simulink model "simscape_robot_delta_v9"  (R2024b)
settings: Solver=FixedStepAuto  StartTime=0.0  StopTime=20.0  FixedStep=1e-6  RelTol=1e-3
model workspace (MAT data in the model file):
  Ts = 1e-06
  kd1 = 14
  kd2 = 13.6
  kd3 = 37.9
  ki1 = 39
  ki2 = 36
  ki3 = 11.6
  kp1 = 12.6
  kp2 = 12.2
  kp3 = 14.4
values from neighbouring files (symbols this model uses):
  N = floor(size(err,1)/window)    [grafica_error.m]
undefined symbols (not defined in the file or in its folder): DiscIntNeverNeededParam, X, Y, Z
libraries: sm_lib x81, nesl_utility x7, spsUniversalBridgeLib x6, spsCurrentMeasurementLib x6, spsDCVoltageSourceLib x3, spsStepperMotorLib x3, spspowerguiLib x1
(part 1 of 3)
settings Model: Creator=rodri  LastModifiedBy=rodri

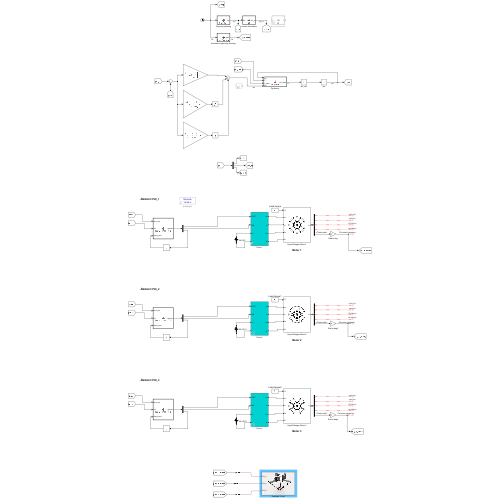
[thumbnail: Simulink's stored preview of the top-level diagram]
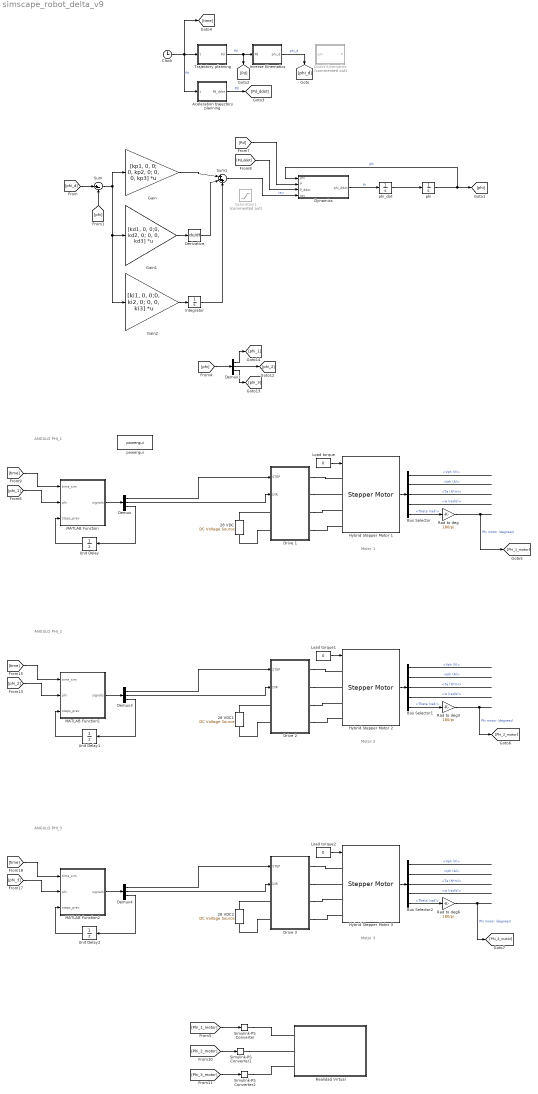
== system simscape_robot_delta_v9 ==
  note: Motor 3
  note: ÁNGULO PHI_1
  note: Motor 1
  note: ÁNGULO PHI_2
  note: ÁNGULO PHI_3
  note: Motor 2
  28 VDC : spsDCVoltageSourceLib/DC Voltage Source  Amplitude=28  Measurements=None
  28 VDC1 : spsDCVoltageSourceLib/DC Voltage Source  Amplitude=28  Measurements=None
  28 VDC2 : spsDCVoltageSourceLib/DC Voltage Source  Amplitude=28  Measurements=None
  Aceleration trajectory planning : MATLAB Function  TreatAsAtomicUnit=on
  Bus Selector : BusSelector  OutputSignals=Vph (V),Iph (A),Te (N*m),w (rad/s),Theta (rad)
  Bus Selector1 : BusSelector  OutputSignals=Vph (V),Iph (A),Te (N*m),w (rad/s),Theta (rad)
  Bus Selector2 : BusSelector  OutputSignals=Vph (V),Iph (A),Te (N*m),w (rad/s),Theta (rad)
  Clock : Clock
  Demux{,1,3..4} (4 alike) : Demux  Outputs=3
  Derivative : Derivative
  Direct Kinematics : MATLAB Function  Commented=on  TreatAsAtomicUnit=on
  Drive 1 : Subsystem  mask{Iref=2, step=500, Ts=Ts}
      mask prompts: Iref "Phase current (A)"; step "Stepping rate (step/s)"; Ts "Sampling time (s)"
      mask init:
      | Nstep=round(1/step/Ts);
  Drive 2 : Subsystem  mask{Iref=2, step=500, Ts=Ts}
      mask prompts: Iref "Phase current (A)"; step "Stepping rate (step/s)"; Ts "Sampling time (s)"
      mask init:
      | Nstep=round(1/step/Ts);
  Drive 3 : Subsystem  mask{Iref=2, step=500, Ts=Ts}
      mask prompts: Iref "Phase current (A)"; step "Stepping rate (step/s)"; Ts "Sampling time (s)"
      mask init:
      | Nstep=round(1/step/Ts);
  Dynamics : MATLAB Function  TreatAsAtomicUnit=on
  Gain : Gain  Gain=[kp1, 0, 0; 0, kp2, 0; 0, 0, kp3]  Multiplication=Matrix(K*u)
  Gain1 : Gain  Gain=[kd1, 0, 0;0, kd2, 0; 0, 0, kd3]  Multiplication=Matrix(K*u)
  Gain2 : Gain  Gain=[ki1, 0, 0;0, ki2, 0; 0, 0, ki3]  Multiplication=Matrix(K*u)
  Hybrid Stepper Motor 1 : spsStepperMotorLib/Stepper Motor  MotorType=Permanent-magnet / Hybrid  NumberOfPhases_1=2  NumberOfPhases_2=3  PresetModel_1=<empty>  PresetModel_2=<empty>  L=1.4e-3  Lmax=10e-3  Lmin=2e-3  R=0.7  Step_angle=1.8  Psim=0.005  Tdm=0.002  J=1.2e-7  B=1e-7*1000  w0=0  pos0=0  TsPowergui=0  TsBlock=-1
  Hybrid Stepper Motor 2 : spsStepperMotorLib/Stepper Motor  MotorType=Permanent-magnet / Hybrid  NumberOfPhases_1=2  NumberOfPhases_2=3  PresetModel_1=<empty>  PresetModel_2=<empty>  L=1.4e-3  Lmax=10e-3  Lmin=2e-3  R=0.7  Step_angle=1.8  Psim=0.005  Tdm=0.002  J=1.2e-7  B=1e-7*1000  w0=0  pos0=0  TsPowergui=0  TsBlock=-1
  Hybrid Stepper Motor 3 : spsStepperMotorLib/Stepper Motor  MotorType=Permanent-magnet / Hybrid  NumberOfPhases_1=2  NumberOfPhases_2=3  PresetModel_1=<empty>  PresetModel_2=<empty>  L=1.4e-3  Lmax=10e-3  Lmin=2e-3  R=0.7  Step_angle=1.8  Psim=0.005  Tdm=0.002  J=1.2e-7  B=1e-7*1000  w0=0  pos0=0  TsPowergui=0  TsBlock=-1
  Integrator : Integrator  InitialCondition=[0;0;0]
  Inverse Kinematics : MATLAB Function  TreatAsAtomicUnit=on
  Load torque : Constant  Value=0
  Load torque1 : Constant  Value=0
  Load torque2 : Constant  Value=0
  MATLAB Function : MATLAB Function  TreatAsAtomicUnit=on
  MATLAB Function1 : MATLAB Function  TreatAsAtomicUnit=on
  MATLAB Function2 : MATLAB Function  TreatAsAtomicUnit=on
  Rad to deg : Gain  Gain=180/pi
  Rad to deg3 : Gain  Gain=180/pi
  Rad to deg6 : Gain  Gain=180/pi
  Realidad Virtual : Subsystem
      mask Display: image('robot_delta_azucena.png');
  Saturation1 : Saturate  Commented=on  UpperLimit=19.8  LowerLimit=-19.8
  Simulink-PS Converter : nesl_utility/Simulink-PS Converter  PhysicalDomain=network_engine_domain  SubClassName=ps_input  LeftPortType=input  RightPortType=output  PseudoPeriodic=off  Frequencies=[]  NoiseDistribution=none  NoiseParameters=[]  Unit=deg  AffineConversion=off  FilteringAndDerivatives=filter  SimscapeFilterOrder=2  InputFilterTimeConstant=0.001  UdotUserProvided=0
  Simulink-PS Converter1 : nesl_utility/Simulink-PS Converter  PhysicalDomain=network_engine_domain  SubClassName=ps_input  LeftPortType=input  RightPortType=output  PseudoPeriodic=off  Frequencies=[]  NoiseDistribution=none  NoiseParameters=[]  Unit=deg  AffineConversion=off  FilteringAndDerivatives=filter  SimscapeFilterOrder=2  InputFilterTimeConstant=0.001  UdotUserProvided=0
  Simulink-PS Converter2 : nesl_utility/Simulink-PS Converter  PhysicalDomain=network_engine_domain  SubClassName=ps_input  LeftPortType=input  RightPortType=output  PseudoPeriodic=off  Frequencies=[]  NoiseDistribution=none  NoiseParameters=[]  Unit=deg  AffineConversion=off  FilteringAndDerivatives=filter  SimscapeFilterOrder=2  InputFilterTimeConstant=0.001  UdotUserProvided=0
  Sum : Sum  Inputs=|+-
  Sum1 : Sum  Inputs=|+++
  Trajectory planning : MATLAB Function  TreatAsAtomicUnit=on
  Unit Delay : UnitDelay  SampleTime=-1  HasFrameUpgradeWarning=on
  Unit Delay1 : UnitDelay  SampleTime=-1  HasFrameUpgradeWarning=on
  Unit Delay2 : UnitDelay  SampleTime=-1  HasFrameUpgradeWarning=on
  phi : Integrator  InitialCondition=[0;0;0]
  phi_dot : Integrator  InitialCondition=[0;0;0]
  powergui : spspowerguiLib/powergui  SimulationMode=Discrete  SampleTime=Ts  frequency=60  Iterations=50  frequencyindice=0  Pbase=100e6  ErrMax=1e-4  UnitsV=kV  UnitsW=MW  buscounter=0  FunctionMessages=off  echomessages=off  EnableUseOfTLC=off  CurrentSourceSwitches=off  DisableSnubberDevices=off  DisableRonSwitches=off  DisableVfSwitches=off  DisplayEquations=off  AutomaticDiscreteSolvers=off  SolverType=Tustin/Backward Euler (TBE)  Interpol=off  ExternalGateDelay=off  methode=off  Ts=0  x0status=blocks  SPID=off  SwTol=0  HookPort=off  NonlinearTolerance=1e-4  nMaxIteration=100  ContinueOnMaxIteration=off  RestoreLinks=warning  ResistiveCurrentMeasurement=off  Frange=[0:2:500]  Ylog=off  Xlog=on  ShowGrid=off  save=off  variable=ZData  structure=0  ZoomFFT=on  StartTime=0.0  cycles=1  DisplayStyle=1  fundamental=60  FreqAxis=off  MaxFrequency=1000  frequencyindicesteady=1  RmsSteady=1  display=off
  wires:
  Sum/1 -> Gain2/1, Gain1/1, Gain/1
  Gain/1 -> Sum1/1
  Derivative/1 -> Sum1/2
  [Pd] -> Dynamics/2(P)
  Clock/1 -> [time], Aceleration trajectory planning/1(t), Trajectory planning/1(t)  "Pd"
  phi/1 -> Dynamics/1(phi), [phi]  "phi"
  Integrator/1 -> Sum1/3
  [Pd_ddot] -> Dynamics/3(P_ddot)
  Sum1/1 -> Dynamics/4(tau)  "tau"
  Gain1/1 -> Derivative/1
  [phi_d] -> Sum/1
  Trajectory planning/1(Pd) -> Inverse Kinematics/1(Pd), [Pd]  "Pd"
  Dynamics/1(phi_ddot) -> phi_dot/1  "Pr"
  Gain2/1 -> Integrator/1
  phi_dot/1 -> phi/1
  Inverse Kinematics/1(phi_d) -> [phi_d]  "phi_d"
  Aceleration trajectory planning/1(Pd_ddot) -> [Pd_ddot]  "Pd"
  [phi] -> Sum/2
  Bus Selector/1 -> ?  "<Vph (V)>"
  Load torque/1 -> Hybrid Stepper Motor 1/1
  [phi_2] -> MATLAB Function1/2(phi)
  Demux3/3 -> Unit Delay1/1
  [time] -> MATLAB Function/1(time_sim)
  [time] -> MATLAB Function1/1(time_sim)
  Bus Selector/5 -> Rad to deg/1  "<Theta (rad)>"
  Bus Selector/4 -> ?  "<w (rad/s)>"
  Demux/3 -> Unit Delay/1
  Hybrid Stepper Motor 2/1 -> Bus Selector1/1
  Rad to deg/1 -> [Phi_1_motor]  "Phi motor (degrees)"
  Demux/2 -> Drive 1/2(DIR)
  Bus Selector2/3 -> ?  "<Te (N*m)>"
  Rad to deg6/1 -> [Phi_3_motor]  "Phi motor (degrees)"
  Unit Delay2/1 -> MATLAB Function2/3(steps_prev)
  Bus Selector2/2 -> ?  "<Iph (A)>"
  Unit Delay1/1 -> MATLAB Function1/3(steps_prev)
  Bus Selector2/4 -> ?  "<w (rad/s)>"
  Hybrid Stepper Motor 1/1 -> Bus Selector/1
  Bus Selector2/5 -> Rad to deg6/1  "<Theta (rad)>"
  Load torque1/1 -> Hybrid Stepper Motor 2/1
  MATLAB Function1/1(signals) -> Demux3/1
  Load torque2/1 -> Hybrid Stepper Motor 3/1
  Demux4/3 -> Unit Delay2/1
  Demux3/2 -> Drive 2/2(DIR)
  [phi_3] -> MATLAB Function2/2(phi)
  Demux/1 -> Drive 1/1(STEP)
  Bus Selector2/1 -> ?  "<Vph (V)>"
  Bus Selector1/4 -> ?  "<w (rad/s)>"
  Bus Selector/3 -> ?  "<Te (N*m)>"
  Demux4/1 -> Drive 3/1(STEP)
  Bus Selector1/5 -> Rad to deg3/1  "<Theta (rad)>"
  Hybrid Stepper Motor 3/1 -> Bus Selector2/1
  Bus Selector/2 -> ?  "<Iph (A)>"
  Bus Selector1/1 -> ?  "<Vph (V)>"
  [phi_1] -> MATLAB Function/2(phi)
  Demux4/2 -> Drive 3/2(DIR)
  Bus Selector1/3 -> ?  "<Te (N*m)>"
  MATLAB Function/1(signals) -> Demux/1
  Rad to deg3/1 -> [Phi_2_motor]  "Phi motor (degrees)"
  [time] -> MATLAB Function2/1(time_sim)
  Demux3/1 -> Drive 2/1(STEP)
  Unit Delay/1 -> MATLAB Function/3(steps_prev)
  MATLAB Function2/1(signals) -> Demux4/1
  Bus Selector1/2 -> ?  "<Iph (A)>"
  Demux1/1 -> [phi_1]
  Demux1/3 -> [phi_3]
  [phi] -> Demux1/1
  Demux1/2 -> [phi_2]
  [Phi_1_motor] -> Simulink-PS Converter/1
  [Phi_2_motor] -> Simulink-PS Converter1/1
  [Phi_3_motor] -> Simulink-PS Converter2/1
  connections:
  Drive 1/RConn2 -- Hybrid Stepper Motor 1/LConn2
  Drive 2/RConn2 -- Hybrid Stepper Motor 2/LConn2
  Drive 3/RConn2 -- Hybrid Stepper Motor 3/LConn2
  Drive 3/RConn3 -- Hybrid Stepper Motor 3/LConn3
  28 VDC2/RConn1 -- Drive 3/LConn1
  Drive 2/LConn2 -- 28 VDC1/LConn1
  Drive 2/RConn3 -- Hybrid Stepper Motor 2/LConn3
  Drive 1/RConn4 -- Hybrid Stepper Motor 1/LConn4
  Drive 2/RConn4 -- Hybrid Stepper Motor 2/LConn4
  Drive 3/LConn2 -- 28 VDC2/LConn1
  28 VDC/RConn1 -- Drive 1/LConn1
  28 VDC1/RConn1 -- Drive 2/LConn1
  Drive 1/RConn3 -- Hybrid Stepper Motor 1/LConn3
  Drive 1/LConn2 -- 28 VDC/LConn1
  Drive 3/RConn1 -- Hybrid Stepper Motor 3/LConn1
  Drive 1/RConn1 -- Hybrid Stepper Motor 1/LConn1
  Drive 3/RConn4 -- Hybrid Stepper Motor 3/LConn4
  Drive 2/RConn1 -- Hybrid Stepper Motor 2/LConn1
  Simulink-PS Converter2/RConn1 -- Realidad Virtual/LConn3
  Simulink-PS Converter1/RConn1 -- Realidad Virtual/LConn2
  Simulink-PS Converter/RConn1 -- Realidad Virtual/LConn1

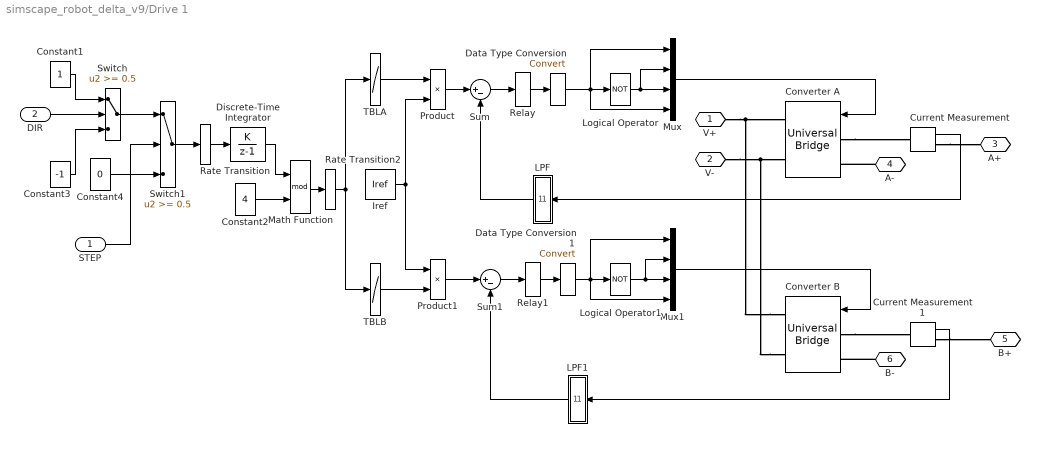
== system simscape_robot_delta_v9/Drive 1 ==
  STEP : Inport
  DIR : Inport  Port=2
  Constant1 : Constant  SampleTime=Ts
  Constant2 : Constant  Value=4  SampleTime=Nstep*Ts
  Constant3 : Constant  Value=-1  SampleTime=Ts
  Constant4 : Constant  Value=0  SampleTime=Ts
  Converter A : spsUniversalBridgeLib/Universal Bridge  Arms=2  SnubberResistance=10000  SnubberCapacitance=inf  Device=MOSFET / Diodes  Ron=1e-3*10  Lon=0  ForwardVoltages="[  0  0  ]"  ForwardVoltage=0  GTOparameters=[ 10e-6 , 20e-6 ]  IGBTparameters=[ 0.5e-6 , 0.5e-6 ]  Measurements=None  Measurements_2=None  converterType=Rectifier
  Converter B : spsUniversalBridgeLib/Universal Bridge  Arms=2  SnubberResistance=10000  SnubberCapacitance=inf  Device=MOSFET / Diodes  Ron=1e-3*10  Lon=0  ForwardVoltages="[  0  0  ]"  ForwardVoltage=0  GTOparameters=[ 10e-6 , 20e-6 ]  IGBTparameters=[ 0.5e-6 , 0.5e-6 ]  Measurements=None  Measurements_2=None  converterType=Rectifier
  Current Measurement : spsCurrentMeasurementLib/Current Measurement  PhasorSimulation=off  OutputType=Complex  PSBequivalent=0
  Current Measurement1 : spsCurrentMeasurementLib/Current Measurement  PhasorSimulation=off  OutputType=Complex  PSBequivalent=0
  Data Type Conversion : DataTypeConversion  SaturateOnIntegerOverflow=off  RndMeth=Floor
  Data Type Conversion1 : DataTypeConversion  SaturateOnIntegerOverflow=off  RndMeth=Floor
  Discrete-Time Integrator : DiscreteIntegrator  IntegratorMethod=Accumulation: Forward Euler  SampleTime=Nstep*Ts  ICPrevOutput=DiscIntNeverNeededParam  ICPrevScaledInput=DiscIntNeverNeededParam
  Iref : Constant  Value=Iref  SampleTime=Ts
  LPF : Subsystem  mask{fc=10000, Ts=Ts}
      mask prompts: fc "Cut-off frequency (Hz)"; Ts "Sampling time (s)"
      mask init:
      | % fa=tf(1,[1/2/pi/fc 1]);
      | % fn=c2d(fa,Ts);
      | % [NN,DD]=tfdata(fn,'v')
      | 
      | NN = [ 0,0.0609];
      | DD = [1.0000,-0.9391];
  LPF1 : Subsystem  mask{fc=10000, Ts=Ts}
      mask prompts: fc "Cut-off frequency (Hz)"; Ts "Sampling time (s)"
      mask init:
      | % fa=tf(1,[1/2/pi/fc 1]);
      | % fn=c2d(fa,Ts);
      | % [NN,DD]=tfdata(fn,'v')
      | 
      | NN = [ 0,0.0609];
      | DD = [1.0000,-0.9391];
  Logical Operator : Logic  Operator=NOT  AllPortsSameDT=off  OutDataTypeStr=boolean
  Logical Operator1 : Logic  Operator=NOT  AllPortsSameDT=off  OutDataTypeStr=boolean
  Math Function : Math  Operator=mod  SignedPower=on  SampleTime=Nstep*Ts
  Mux : Mux
  Mux1 : Mux
  Product : Product  RndMeth=Zero
  Product1 : Product  RndMeth=Zero
  Rate Transition : RateTransition
  Rate Transition2 : RateTransition
  Relay : Relay  OnSwitchValue=0.01  OffSwitchValue=-0.01
  Relay1 : Relay  OnSwitchValue=0.01  OffSwitchValue=-0.01  OutDataTypeStr=Inherit: Inherit via back propagation
  Sum : Sum  Inputs=|+-  OutDataTypeStr=Inherit: Same as first input
  Sum1 : Sum  Inputs=|+-  OutDataTypeStr=Inherit: Same as first input
  Switch : Switch  Threshold=0.5  ZeroCross=off  SampleTime=Ts  SaturateOnIntegerOverflow=off  InputSameDT=off
  Switch1 : Switch  Threshold=0.5  ZeroCross=off  SampleTime=Ts  SaturateOnIntegerOverflow=off  InputSameDT=off
  TBLA : Lookup_n-D  NumberOfTableDimensions=1  BreakpointsForDimension1=[0:3]  BreakpointsForDimension2=[0 571.55 685.8 800.15 914.4 1028.8 1143.1 1257.4 1371.7 1486 1600.3 1714.6 1828.9 1943.2 2057.5 2171.8 2286.1 2400.5 2514.7 2629.1 2743.3 2857.7 2971.9 3086.3 3200.5 3314.9 3429.2]  Table=[1 0 -1 0]  InternalRulePriority=Speed  RndMeth=Simplest
  TBLB : Lookup_n-D  NumberOfTableDimensions=1  BreakpointsForDimension1=[0:3]  BreakpointsForDimension2=[0 571.55 685.8 800.15 914.4 1028.8 1143.1 1257.4 1371.7 1486 1600.3 1714.6 1828.9 1943.2 2057.5 2171.8 2286.1 2400.5 2514.7 2629.1 2743.3 2857.7 2971.9 3086.3 3200.5 3314.9 3429.2]  Table=[0 1 0 -1]  InternalRulePriority=Speed  RndMeth=Simplest
  V+ : PMIOPort  Side=Left
  V- : PMIOPort  Port=2  Side=Left
  A+ : PMIOPort  Port=3  Side=Right
  A- : PMIOPort  Port=4  Side=Right
  B+ : PMIOPort  Port=5  Side=Right
  B- : PMIOPort  Port=6  Side=Right
  wires:
  Constant4/1 -> Switch1/3
  Switch1/1 -> Rate Transition/1
  Switch/1 -> Switch1/1
  STEP/1 -> Switch1/2
  DIR/1 -> Switch/2
  Rate Transition2/1 -> TBLB/1, TBLA/1
  Math Function/1 -> Rate Transition2/1
  Product1/1 -> Sum1/1
  Product/1 -> Sum/1
  Rate Transition/1 -> Discrete-Time Integrator/1
  Constant3/1 -> Switch/3
  Constant1/1 -> Switch/1
  Discrete-Time Integrator/1 -> Math Function/1
  Constant2/1 -> Math Function/2
  Iref/1 -> Product1/1, Product/2
  TBLB/1 -> Product1/2
  TBLA/1 -> Product/1
  LPF1/1(O) -> Sum1/2
  LPF/1(O) -> Sum/2
  Data Type Conversion1/1 -> Mux1/4, Mux1/1, Logical Operator1/1
  Data Type Conversion/1 -> Logical Operator/1, Mux/4, Mux/1
  Current Measurement1/1 -> LPF1/1(I)
  Sum1/1 -> Relay1/1
  Mux1/1 -> Converter B/1
  Logical Operator1/1 -> Mux1/2, Mux1/3
  Relay1/1 -> Data Type Conversion1/1
  Mux/1 -> Converter A/1
  Logical Operator/1 -> Mux/2, Mux/3
  Relay/1 -> Data Type Conversion/1
  Current Measurement/1 -> LPF/1(I)
  Sum/1 -> Relay/1
  connections:
  Converter B/RConn2 -- Converter A/RConn2 -- V-/RConn1
  Converter B/RConn1 -- Converter A/RConn1 -- V+/RConn1
  Current Measurement1/RConn1 -- B+/RConn1
  Converter B/LConn1 -- Current Measurement1/LConn1
  Current Measurement/RConn1 -- A+/RConn1
  Converter A/LConn1 -- Current Measurement/LConn1
  B-/RConn1 -- Converter B/LConn2
  A-/RConn1 -- Converter A/LConn2

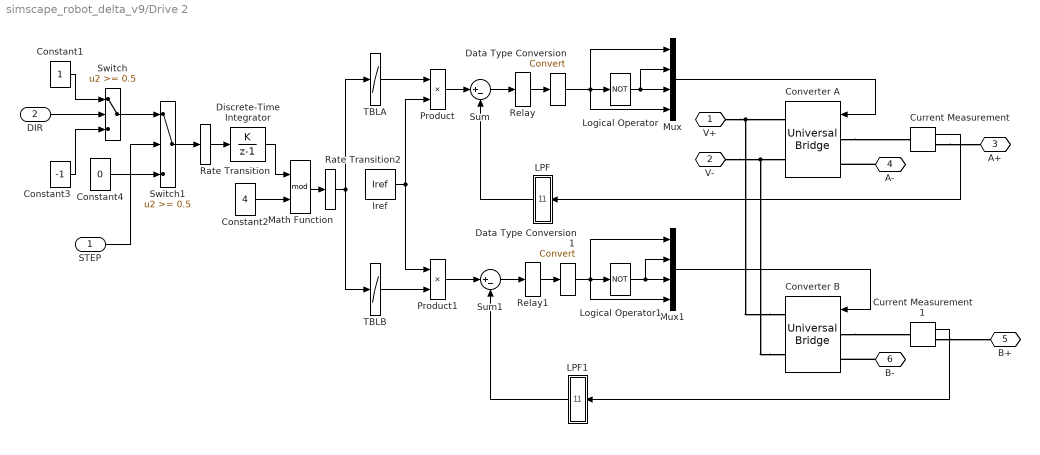
== system simscape_robot_delta_v9/Drive 2 ==
  STEP : Inport
  DIR : Inport  Port=2
  Constant1 : Constant  SampleTime=Ts
  Constant2 : Constant  Value=4  SampleTime=Nstep*Ts
  Constant3 : Constant  Value=-1  SampleTime=Ts
  Constant4 : Constant  Value=0  SampleTime=Ts
  Converter A : spsUniversalBridgeLib/Universal Bridge  Arms=2  SnubberResistance=10000  SnubberCapacitance=inf  Device=MOSFET / Diodes  Ron=1e-3*10  Lon=0  ForwardVoltages="[  0  0  ]"  ForwardVoltage=0  GTOparameters=[ 10e-6 , 20e-6 ]  IGBTparameters=[ 0.5e-6 , 0.5e-6 ]  Measurements=None  Measurements_2=None  converterType=Rectifier
  Converter B : spsUniversalBridgeLib/Universal Bridge  Arms=2  SnubberResistance=10000  SnubberCapacitance=inf  Device=MOSFET / Diodes  Ron=1e-3*10  Lon=0  ForwardVoltages="[  0  0  ]"  ForwardVoltage=0  GTOparameters=[ 10e-6 , 20e-6 ]  IGBTparameters=[ 0.5e-6 , 0.5e-6 ]  Measurements=None  Measurements_2=None  converterType=Rectifier
  Current Measurement : spsCurrentMeasurementLib/Current Measurement  PhasorSimulation=off  OutputType=Complex  PSBequivalent=0
  Current Measurement1 : spsCurrentMeasurementLib/Current Measurement  PhasorSimulation=off  OutputType=Complex  PSBequivalent=0
  Data Type Conversion : DataTypeConversion  SaturateOnIntegerOverflow=off  RndMeth=Floor
  Data Type Conversion1 : DataTypeConversion  SaturateOnIntegerOverflow=off  RndMeth=Floor
  Discrete-Time Integrator : DiscreteIntegrator  IntegratorMethod=Accumulation: Forward Euler  SampleTime=Nstep*Ts  ICPrevOutput=DiscIntNeverNeededParam  ICPrevScaledInput=DiscIntNeverNeededParam
  Iref : Constant  Value=Iref  SampleTime=Ts
  LPF : Subsystem  mask{fc=10000, Ts=Ts}
      mask prompts: fc "Cut-off frequency (Hz)"; Ts "Sampling time (s)"
      mask init:
      | % fa=tf(1,[1/2/pi/fc 1]);
      | % fn=c2d(fa,Ts);
      | % [NN,DD]=tfdata(fn,'v')
      | 
      | NN = [ 0,0.0609];
      | DD = [1.0000,-0.9391];
  LPF1 : Subsystem  mask{fc=10000, Ts=Ts}
      mask prompts: fc "Cut-off frequency (Hz)"; Ts "Sampling time (s)"
      mask init:
      | % fa=tf(1,[1/2/pi/fc 1]);
      | % fn=c2d(fa,Ts);
      | % [NN,DD]=tfdata(fn,'v')
      | 
      | NN = [ 0,0.0609];
      | DD = [1.0000,-0.9391];
  Logical Operator : Logic  Operator=NOT  AllPortsSameDT=off  OutDataTypeStr=boolean
  Logical Operator1 : Logic  Operator=NOT  AllPortsSameDT=off  OutDataTypeStr=boolean
  Math Function : Math  Operator=mod  SignedPower=on  SampleTime=Nstep*Ts
  Mux : Mux
  Mux1 : Mux
  Product : Product  RndMeth=Zero
  Product1 : Product  RndMeth=Zero
  Rate Transition : RateTransition
  Rate Transition2 : RateTransition
  Relay : Relay  OnSwitchValue=0.01  OffSwitchValue=-0.01
  Relay1 : Relay  OnSwitchValue=0.01  OffSwitchValue=-0.01  OutDataTypeStr=Inherit: Inherit via back propagation
  Sum : Sum  Inputs=|+-  OutDataTypeStr=Inherit: Same as first input
  Sum1 : Sum  Inputs=|+-  OutDataTypeStr=Inherit: Same as first input
  Switch : Switch  Threshold=0.5  ZeroCross=off  SampleTime=Ts  SaturateOnIntegerOverflow=off  InputSameDT=off
  Switch1 : Switch  Threshold=0.5  ZeroCross=off  SampleTime=Ts  SaturateOnIntegerOverflow=off  InputSameDT=off
  TBLA : Lookup_n-D  NumberOfTableDimensions=1  BreakpointsForDimension1=[0:3]  BreakpointsForDimension2=[0 571.55 685.8 800.15 914.4 1028.8 1143.1 1257.4 1371.7 1486 1600.3 1714.6 1828.9 1943.2 2057.5 2171.8 2286.1 2400.5 2514.7 2629.1 2743.3 2857.7 2971.9 3086.3 3200.5 3314.9 3429.2]  Table=[1 0 -1 0]  InternalRulePriority=Speed  RndMeth=Simplest
  TBLB : Lookup_n-D  NumberOfTableDimensions=1  BreakpointsForDimension1=[0:3]  BreakpointsForDimension2=[0 571.55 685.8 800.15 914.4 1028.8 1143.1 1257.4 1371.7 1486 1600.3 1714.6 1828.9 1943.2 2057.5 2171.8 2286.1 2400.5 2514.7 2629.1 2743.3 2857.7 2971.9 3086.3 3200.5 3314.9 3429.2]  Table=[0 1 0 -1]  InternalRulePriority=Speed  RndMeth=Simplest
  V+ : PMIOPort  Side=Left
  V- : PMIOPort  Port=2  Side=Left
  A+ : PMIOPort  Port=3  Side=Right
  A- : PMIOPort  Port=4  Side=Right
  B+ : PMIOPort  Port=5  Side=Right
  B- : PMIOPort  Port=6  Side=Right
  wires:
  Constant4/1 -> Switch1/3
  Switch1/1 -> Rate Transition/1
  Switch/1 -> Switch1/1
  STEP/1 -> Switch1/2
  DIR/1 -> Switch/2
  Rate Transition2/1 -> TBLB/1, TBLA/1
  Math Function/1 -> Rate Transition2/1
  Product1/1 -> Sum1/1
  Product/1 -> Sum/1
  Rate Transition/1 -> Discrete-Time Integrator/1
  Constant3/1 -> Switch/3
  Constant1/1 -> Switch/1
  Discrete-Time Integrator/1 -> Math Function/1
  Constant2/1 -> Math Function/2
  Iref/1 -> Product1/1, Product/2
  TBLB/1 -> Product1/2
  TBLA/1 -> Product/1
  LPF1/1(O) -> Sum1/2
  LPF/1(O) -> Sum/2
  Data Type Conversion1/1 -> Mux1/4, Mux1/1, Logical Operator1/1
  Data Type Conversion/1 -> Logical Operator/1, Mux/4, Mux/1
  Current Measurement1/1 -> LPF1/1(I)
  Sum1/1 -> Relay1/1
  Mux1/1 -> Converter B/1
  Logical Operator1/1 -> Mux1/2, Mux1/3
  Relay1/1 -> Data Type Conversion1/1
  Mux/1 -> Converter A/1
  Logical Operator/1 -> Mux/2, Mux/3
  Relay/1 -> Data Type Conversion/1
  Current Measurement/1 -> LPF/1(I)
  Sum/1 -> Relay/1
  connections:
  Converter B/RConn2 -- Converter A/RConn2 -- V-/RConn1
  Converter B/RConn1 -- Converter A/RConn1 -- V+/RConn1
  Current Measurement1/RConn1 -- B+/RConn1
  Converter B/LConn1 -- Current Measurement1/LConn1
  Current Measurement/RConn1 -- A+/RConn1
  Converter A/LConn1 -- Current Measurement/LConn1
  B-/RConn1 -- Converter B/LConn2
  A-/RConn1 -- Converter A/LConn2

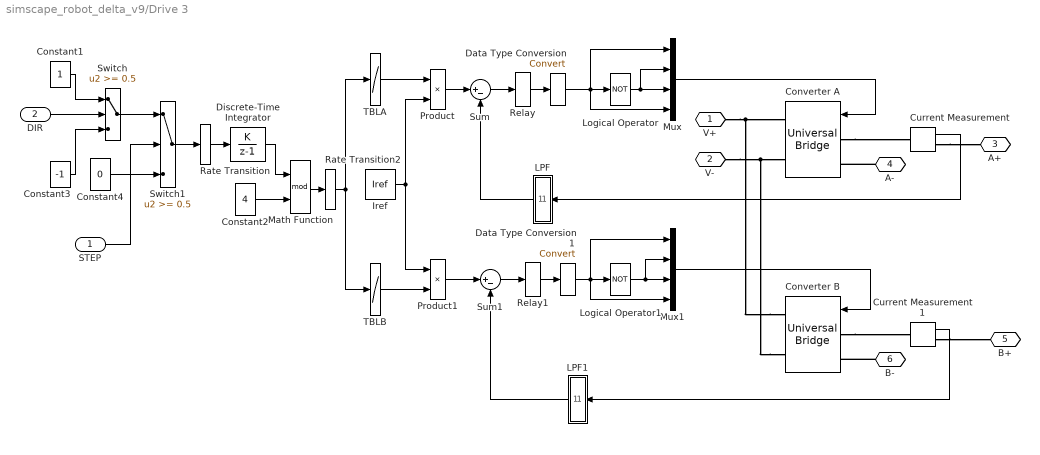
== system simscape_robot_delta_v9/Drive 3 ==
  STEP : Inport
  DIR : Inport  Port=2
  Constant1 : Constant  SampleTime=Ts
  Constant2 : Constant  Value=4  SampleTime=Nstep*Ts
  Constant3 : Constant  Value=-1  SampleTime=Ts
  Constant4 : Constant  Value=0  SampleTime=Ts
  Converter A : spsUniversalBridgeLib/Universal Bridge  Arms=2  SnubberResistance=10000  SnubberCapacitance=inf  Device=MOSFET / Diodes  Ron=1e-3*10  Lon=0  ForwardVoltages="[  0  0  ]"  ForwardVoltage=0  GTOparameters=[ 10e-6 , 20e-6 ]  IGBTparameters=[ 0.5e-6 , 0.5e-6 ]  Measurements=None  Measurements_2=None  converterType=Rectifier
  Converter B : spsUniversalBridgeLib/Universal Bridge  Arms=2  SnubberResistance=10000  SnubberCapacitance=inf  Device=MOSFET / Diodes  Ron=1e-3*10  Lon=0  ForwardVoltages="[  0  0  ]"  ForwardVoltage=0  GTOparameters=[ 10e-6 , 20e-6 ]  IGBTparameters=[ 0.5e-6 , 0.5e-6 ]  Measurements=None  Measurements_2=None  converterType=Rectifier
  Current Measurement : spsCurrentMeasurementLib/Current Measurement  PhasorSimulation=off  OutputType=Complex  PSBequivalent=0
  Current Measurement1 : spsCurrentMeasurementLib/Current Measurement  PhasorSimulation=off  OutputType=Complex  PSBequivalent=0
  Data Type Conversion : DataTypeConversion  SaturateOnIntegerOverflow=off  RndMeth=Floor
  Data Type Conversion1 : DataTypeConversion  SaturateOnIntegerOverflow=off  RndMeth=Floor
  Discrete-Time Integrator : DiscreteIntegrator  IntegratorMethod=Accumulation: Forward Euler  SampleTime=Nstep*Ts  ICPrevOutput=DiscIntNeverNeededParam  ICPrevScaledInput=DiscIntNeverNeededParam
  Iref : Constant  Value=Iref  SampleTime=Ts
  LPF : Subsystem  mask{fc=10000, Ts=Ts}
      mask prompts: fc "Cut-off frequency (Hz)"; Ts "Sampling time (s)"
      mask init:
      | % fa=tf(1,[1/2/pi/fc 1]);
      | % fn=c2d(fa,Ts);
      | % [NN,DD]=tfdata(fn,'v')
      | 
      | NN = [ 0,0.0609];
      | DD = [1.0000,-0.9391];
  LPF1 : Subsystem  mask{fc=10000, Ts=Ts}
      mask prompts: fc "Cut-off frequency (Hz)"; Ts "Sampling time (s)"
      mask init:
      | % fa=tf(1,[1/2/pi/fc 1]);
      | % fn=c2d(fa,Ts);
      | % [NN,DD]=tfdata(fn,'v')
      | 
      | NN = [ 0,0.0609];
      | DD = [1.0000,-0.9391];
  Logical Operator : Logic  Operator=NOT  AllPortsSameDT=off  OutDataTypeStr=boolean
  Logical Operator1 : Logic  Operator=NOT  AllPortsSameDT=off  OutDataTypeStr=boolean
  Math Function : Math  Operator=mod  SignedPower=on  SampleTime=Nstep*Ts
  Mux : Mux
  Mux1 : Mux
  Product : Product  RndMeth=Zero
  Product1 : Product  RndMeth=Zero
  Rate Transition : RateTransition
  Rate Transition2 : RateTransition
  Relay : Relay  OnSwitchValue=0.01  OffSwitchValue=-0.01
  Relay1 : Relay  OnSwitchValue=0.01  OffSwitchValue=-0.01  OutDataTypeStr=Inherit: Inherit via back propagation
  Sum : Sum  Inputs=|+-  OutDataTypeStr=Inherit: Same as first input
  Sum1 : Sum  Inputs=|+-  OutDataTypeStr=Inherit: Same as first input
  Switch : Switch  Threshold=0.5  ZeroCross=off  SampleTime=Ts  SaturateOnIntegerOverflow=off  InputSameDT=off
  Switch1 : Switch  Threshold=0.5  ZeroCross=off  SampleTime=Ts  SaturateOnIntegerOverflow=off  InputSameDT=off
  TBLA : Lookup_n-D  NumberOfTableDimensions=1  BreakpointsForDimension1=[0:3]  BreakpointsForDimension2=[0 571.55 685.8 800.15 914.4 1028.8 1143.1 1257.4 1371.7 1486 1600.3 1714.6 1828.9 1943.2 2057.5 2171.8 2286.1 2400.5 2514.7 2629.1 2743.3 2857.7 2971.9 3086.3 3200.5 3314.9 3429.2]  Table=[1 0 -1 0]  InternalRulePriority=Speed  RndMeth=Simplest
  TBLB : Lookup_n-D  NumberOfTableDimensions=1  BreakpointsForDimension1=[0:3]  BreakpointsForDimension2=[0 571.55 685.8 800.15 914.4 1028.8 1143.1 1257.4 1371.7 1486 1600.3 1714.6 1828.9 1943.2 2057.5 2171.8 2286.1 2400.5 2514.7 2629.1 2743.3 2857.7 2971.9 3086.3 3200.5 3314.9 3429.2]  Table=[0 1 0 -1]  InternalRulePriority=Speed  RndMeth=Simplest
  V+ : PMIOPort  Side=Left
  V- : PMIOPort  Port=2  Side=Left
  A+ : PMIOPort  Port=3  Side=Right
  A- : PMIOPort  Port=4  Side=Right
  B+ : PMIOPort  Port=5  Side=Right
  B- : PMIOPort  Port=6  Side=Right
  wires:
  Constant4/1 -> Switch1/3
  Switch1/1 -> Rate Transition/1
  Switch/1 -> Switch1/1
  STEP/1 -> Switch1/2
  DIR/1 -> Switch/2
  Rate Transition2/1 -> TBLB/1, TBLA/1
  Math Function/1 -> Rate Transition2/1
  Product1/1 -> Sum1/1
  Product/1 -> Sum/1
  Rate Transition/1 -> Discrete-Time Integrator/1
  Constant3/1 -> Switch/3
  Constant1/1 -> Switch/1
  Discrete-Time Integrator/1 -> Math Function/1
  Constant2/1 -> Math Function/2
  Iref/1 -> Product1/1, Product/2
  TBLB/1 -> Product1/2
  TBLA/1 -> Product/1
  LPF1/1(O) -> Sum1/2
  LPF/1(O) -> Sum/2
  Data Type Conversion1/1 -> Mux1/4, Mux1/1, Logical Operator1/1
  Data Type Conversion/1 -> Logical Operator/1, Mux/4, Mux/1
  Current Measurement1/1 -> LPF1/1(I)
  Sum1/1 -> Relay1/1
  Mux1/1 -> Converter B/1
  Logical Operator1/1 -> Mux1/2, Mux1/3
  Relay1/1 -> Data Type Conversion1/1
  Mux/1 -> Converter A/1
  Logical Operator/1 -> Mux/2, Mux/3
  Relay/1 -> Data Type Conversion/1
  Current Measurement/1 -> LPF/1(I)
  Sum/1 -> Relay/1
  connections:
  Converter B/RConn2 -- Converter A/RConn2 -- V-/RConn1
  Converter B/RConn1 -- Converter A/RConn1 -- V+/RConn1
  Current Measurement1/RConn1 -- B+/RConn1
  Converter B/LConn1 -- Current Measurement1/LConn1
  Current Measurement/RConn1 -- A+/RConn1
  Converter A/LConn1 -- Current Measurement/LConn1
  B-/RConn1 -- Converter B/LConn2
  A-/RConn1 -- Converter A/LConn2
